simulink subsystem "RobotPlant"  (R2022b)
settings: Solver=VariableStepAuto  StartTime=0.0  StopTime=10.0  RelTol=1e-3
settings Model: Creator=Sahil Gaurkar  LastModifiedBy=Sahil Gaurkar

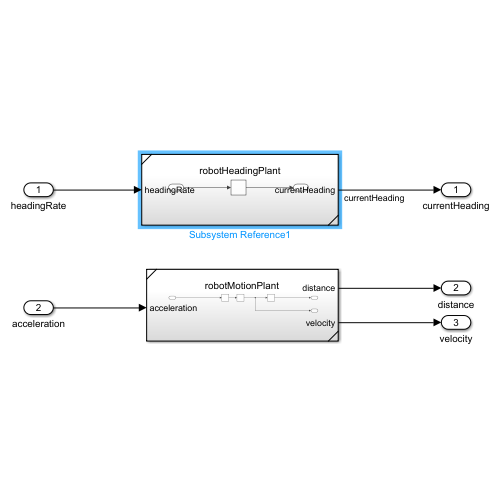
[thumbnail: Simulink's stored preview of the top-level diagram]
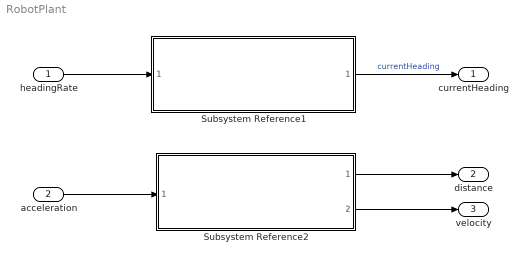
== system RobotPlant ==
  headingRate : Inport
  acceleration : Inport  Port=2
  Subsystem Reference1 : Subsystem  ReferencedSubsystem=robotHeadingPlant
  Subsystem Reference2 : Subsystem  ReferencedSubsystem=robotMotionPlant
  currentHeading : Outport
  distance : Outport  Port=2
  velocity : Outport  Port=3
  wires:
  headingRate/1 -> Subsystem Reference1/1
  acceleration/1 -> Subsystem Reference2/1
  Subsystem Reference1/1 -> currentHeading/1  "currentHeading"
  Subsystem Reference2/2 -> velocity/1
  Subsystem Reference2/1 -> distance/1
